simulink model "PV_with_boost_converter"  (R2018b)
settings: Solver=FixedStepDiscrete  StartTime=0.0  StopTime=3  RelTol=1e-3
undefined symbols (not defined in the file): L, sigbuilder_block
libraries: powerlib x11, re_lib x1, powerlib_meascontrol x1
settings Model: Creator=jetha  LastModifiedBy=jetha

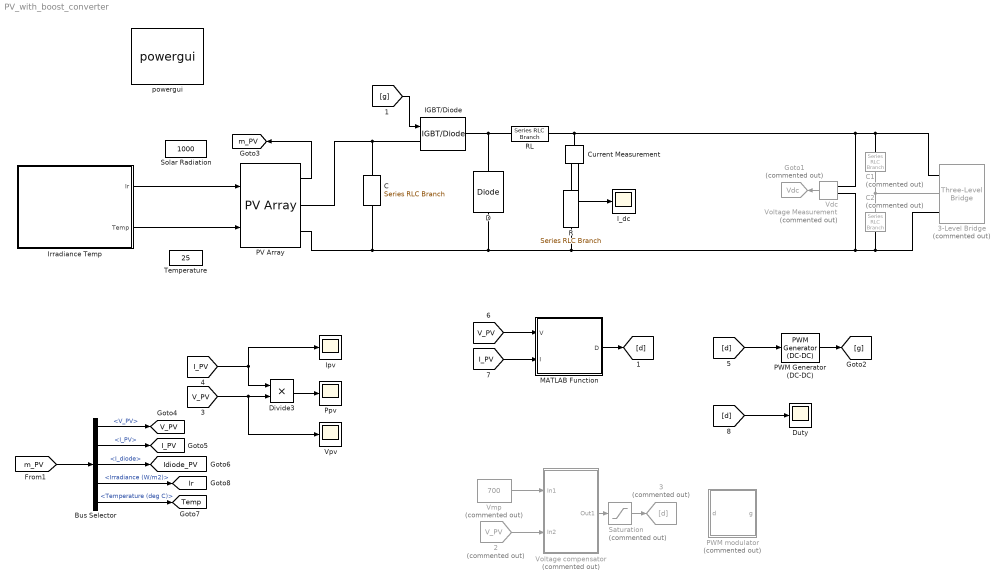
== system PV_with_boost_converter ==
  "       3" : Goto  Commented=on  GotoTag=d
  "   2" : From  Commented=on  GotoTag=V_PV  TagVisibility=global
      settings: CloseFcn=tagdialog Close
  3-Level Bridge : powerlib/Power Electronics/Three-Level Bridge  Commented=on  Arms=3  SnubberResistance=1e6  SbubberCapacitance=inf  Device=IGBT / Diodes  Ron=0.2e-3  ForwardVoltages="[  0  0 ]"  Measurements=None
      settings: SourceProductName=Simscape Electrical  SourceProductBaseCode=PS
  Bus Selector : BusSelector  OutputSignals=V_PV,I_PV,I_diode,Irradiance (W/m2),Temperature (deg C)
  C : powerlib/Elements/Series RLC Branch  LConnTagsString=__new0  RConnTagsString=__new0  BranchType=C  Resistance=1  Inductance=L  SetiL0=off  InitialCurrent=0  Capacitance=10e-3  Setx0=off  InitialVoltage=Vmp  Measurements=None
      settings: SourceProductName=Simscape Electrical
  C1 : powerlib/Elements/Series RLC Branch  Commented=on  LConnTagsString=__new0  RConnTagsString=__new0  BranchType=C  Resistance=1.0  Inductance=1.0  SetiL0=off  InitialCurrent=0  Capacitance=12e-3  Setx0=off  InitialVoltage=0  Measurements=None
      settings: SourceProductName=Simscape Electrical
  C2 : powerlib/Elements/Series RLC Branch  Commented=on  LConnTagsString=__new0  RConnTagsString=__new0  BranchType=C  Resistance=1.0  Inductance=1.0  SetiL0=off  InitialCurrent=0  Capacitance=12e-3  Setx0=off  InitialVoltage=0  Measurements=None
      settings: SourceProductName=Simscape Electrical
  Current Measurement : powerlib/Measurements/Current Measurement  PhasorSimulation=off  OutputType=Complex  PSBequivalent=0
  D : powerlib/Power Electronics/Diode  Ron=1e-4  Lon=0  Vf=0  IC=0  UseSnubber=off  Rs=inf  Cs=inf  Measurements=off
      settings: SourceProductName=Simscape Electrical
  Divide3 : Product  Inputs=**
  Duty : Scope
  Goto1 : Goto  Commented=on  GotoTag=Vdc  TagVisibility=global
  IGBT/Diode : powerlib/Power Electronics/IGBT//Diode  Ron=1e-3  Rs=1e5  Cs=inf  Measurements=off
  I_dc : Scope
  Ipv : Scope
  Irradiance Temp : Subsystem  Tag=STV Subsys  LoadFcn=sigbuilder_block('load');  StartFcn=sigbuilder_block('start');  StopFcn=sigbuilder_block('stop');  ClipboardFcn=sigbuilder_block('clipboard');  mask(Sigbuilder block){tuvar=[0:10]}
      mask help: Sigbuilder GUI
      mask init:
      | if ~strcmp(get_param(bdroot(gcbh),'SimulationStatus'),'stopped') tuvar = sigbuilder_block('maskInit'); end
      settings: CopyFcn=sigbuilder_block('copy');  DeleteFcn=sigbuilder_block('delete');  ModelCloseFcn=sigbuilder_block('modelClose');  PreSaveFcn=sigbuilder_block('preSave');  PauseFcn=sigbuilder_block('pause')  ContinueFcn=sigbuilder_block('continue')  NameChangeFcn=sigbuilder_block('namechange');  OpenFcn=sigbuilder_block('open',[216.75 153.75 550.5 395.25 ]);  CloseFcn=sigbuilder_block('close');
      mask Display: plot(0, 0, 100, 100,[2, 2, 32, 32, 2], [68, 8, 8, 68, 68],[32, 2], [38, 38], [32, 19, 2],[53, 60, 44], [32, 17, 17, 2],[16, 16, 31, 31]);txt = getActiveGroup(gcbh);text(2, 100, txt,'verticalAlignment', 'top');
  MATLAB Function : MATLAB Function  TreatAsAtomicUnit=on
  PV Array : re_lib/Solar/PV Array  Npar=4  Nser=20  PlotType=array @ 1000 W/m2 & specified temperatures  S_vec="[ 1000  500  100 ]"  Temp_C_vec="[ 25  50]"  ModuleName=Waaree Energies WSM-315  PlotWhenSelected=off  Pm=315  Ncell=72  Voc=43  Isc=9.77  Vm=35  Im=9  beta_Voc_pc=-0.338  alpha_Isc_pc=0.040901  beta_Voc=-0.14534  alpha_Isc=0.003996  IL=9.7966  I0=1.447e-10  nI=0.93356  Rsh=115.0566  Rs=0.31273  BAL=off  Tc=1e-6  Tfilter=5e-6
  PWM modulator : Subsystem  Commented=on
  PWM Generator (DC-DC) : powerlib_meascontrol/Pulse & Signal Generators/PWM Generator (DC-DC)  Fsw=10000  Ts=0
  Ppv : Scope
  R : powerlib/Elements/Series RLC Branch  LConnTagsString=__new0  RConnTagsString=__new0  BranchType=R  Resistance=5  Inductance=5e-3  SetiL0=off  InitialCurrent=0  Capacitance=1e-6  Setx0=off  InitialVoltage=0  Measurements=None
      settings: SourceProductName=Simscape Electrical
  RL : powerlib/Elements/Series RLC Branch  LConnTagsString=__new0  RConnTagsString=__new0  BranchType=RL  Resistance=5e-3  Inductance=10e-3  SetiL0=off  InitialCurrent=0  Capacitance=1e-6  Setx0=off  InitialVoltage=0  Measurements=None
      settings: SourceProductName=Simscape Electrical
  Saturation : Saturate  Commented=on  UpperLimit=1  LowerLimit=0
  Solar Radiation : Constant  Value=1000
  Temperature : Constant  Value=25
  "Vdc " : powerlib/Measurements/Voltage Measurement  Tag=PoWeRsYsTeMmEaSuReMeNt  Commented=on  PhasorSimulation=off  OutputType=Magnitude  PSBequivalent=0
      settings: SourceProductName=Simscape Electrical
  Vmp : Constant  Commented=on  Value=700
  Voltage compensator : Subsystem  Commented=on
  Vpv : Scope
  powergui : powerlib/powergui  Priority=1  SimulationMode=Discrete  SampleTime=5e-7  frequency=60  Iterations=50  frequencyindice=0  Pbase=100e6  ErrMax=1e-4  UnitsV=kV  UnitsW=MW  buscounter=0  FunctionMessages=off  echomessages=off  EnableUseOfTLC=off  CurrentSourceSwitches=off  DisableSnubberDevices=off  DisableRonSwitches=off  DisableVfSwitches=off  DisplayEquations=off  SolverType=Tustin/Backward Euler (TBE)  Interpol=off  ExternalGateDelay=off  methode=off  Ts=100  x0status=blocks  SPID=off  SwTol=0  HookPort=off  RestoreLinks=warning  ResistiveCurrentMeasurement=off  Frange=[0:2:500]  Ylog=off  Xlog=on  ShowGrid=off  save=off  variable=ZData  structure=0  ZoomFFT=off  StartTime=0.0  cycles=1  DisplayStyle=1  fundamental=60  FreqAxis=off  MaxFrequency=1000  frequencyindicesteady=1  RmsSteady=1  display=off
  tag scope: I_PV=global, Idiode_PV=global, Ir=global, Temp=global, V_PV=global, m_PV=global
  wires:
  Divide3/1 -> Ppv/1
  [I_PV] -> Ipv/1, Divide3/1
  [V_PV] -> Divide3/2, Vpv/1
  Voltage compensator/1(Out1) -> Saturation/1
  PWM Generator (DC-DC)/1 -> [g]
  "   2"/1 -> Voltage compensator/2(In2)
  [d] -> PWM Generator (DC-DC)/1
  PV Array/1 -> [m_PV]
  Bus Selector/3 -> [Idiode_PV]  "<I_diode>"
  Bus Selector/4 -> [Ir]  "<Irradiance (W/m2)>"
  Bus Selector/1 -> [V_PV]  "<V_PV>"
  Bus Selector/5 -> [Temp]  "<Temperature (deg C)>"
  Bus Selector/2 -> [I_PV]  "<I_PV>"
  [m_PV] -> Bus Selector/1
  "Vdc "/1 -> Goto1/1
  [g] -> IGBT/Diode/1
  Saturation/1 -> "       3"/1
  Current Measurement/1 -> I_dc/1
  [V_PV] -> MATLAB Function/1(V)
  [I_PV] -> MATLAB Function/2(I)
  MATLAB Function/1(D) -> [d]
  Vmp/1 -> Voltage compensator/1(In1)
  [d] -> Duty/1
  Irradiance Temp/1(Ir) -> PV Array/1
  Irradiance Temp/2(Temp) -> PV Array/2
  connections:
  C2/RConn1 -- 3-Level Bridge/RConn3 -- "Vdc "/LConn2 -- R/RConn1 -- C/RConn1 -- PV Array/RConn2 -- D/LConn1
  RL/LConn1 -- Current Measurement/LConn1 -- C1/LConn1 -- 3-Level Bridge/RConn1 -- "Vdc "/LConn1
  3-Level Bridge/RConn2 -- C1/RConn1 -- C2/LConn1
  R/LConn1 -- Current Measurement/RConn1
  D/RConn1 -- IGBT/Diode/RConn1 -- RL/RConn1
  PV Array/RConn1 -- C/LConn1 -- IGBT/Diode/LConn1

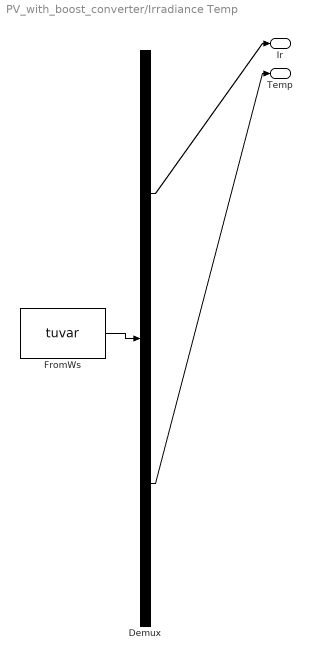
== system PV_with_boost_converter/Irradiance Temp ==
  Demux : Demux  Tag=STV Demux  Outputs=2
  FromWs : FromWorkspace  Tag=STV FromWs  VariableName=tuvar  SampleTime=0
      SigBuilderData=|
      | common.afterFinalStr = 'Extrapolate'
      | common.sampleTime = '0'
      | dataSet(1).timeRange = [0 1]
      | dataSet(1).name = 'Constant Irradiance'
      | dataSet(2).timeRange = [0 1]
      | dataSet(2).name = 'Step Irradiance'
      | dataSet(3).timeRange = [0 3]
      | dataSet(3).name = 'Ramp-up/down Irradiance'
      | sbobj.Groups(1).Name = 'Constant Irradiance'
      | sbobj.Groups(1).Signals(1).Name = 'Ir'
      | sbobj.Groups(1).Signals(1).XData = [0 1]
      | sbobj.Groups(1).Signals(1).YData = [1000 1000]
      | sbobj.Groups(1).Signals(2).Name = 'Temp'
      | sbobj.Groups(1).Signals(2).XData = [0 1 1 2]
      | sbobj.Groups(1).Signals(2).YData = [0 0 1 1]
      | sbobj.Groups(1).TimeRange = [0 1]
      | sbobj.Groups(2).Name = 'Step Irradiance'
      | sbobj.Groups(2).Signals(1).Name = 'Ir'
      | sbobj.Groups(2).Signals(1).XData = [0 0.252 0.252 1]
      | sbobj.Groups(2).Signals(1).YData = [600 600 1000 1000]
      | sbobj.Groups(2).Signals(2).Name = 'Temp'
      | sbobj.Groups(2).Signals(2).XData = [0 1 1 2]
      | sbobj.Groups(2).Signals(2).YData = [0 0 1 1]
      | sbobj.Groups(2).TimeRange = [0 1]
      | sbobj.Groups(3).Name = 'Ramp-up/down Irradiance'
      | sbobj.Groups(3).Signals(1).Name = 'Ir'
      | sbobj.Groups(3).Signals(1).XData = [0 0.6 1.1 1.2 1.7 3]
      | sbobj.Groups(3).Signals(1).YData = [1000 1000 250 250 1000 1000]
      | sbobj.Groups(3).Signals(2).Name = 'Temp'
      | sbobj.Groups(3).Signals(2).XData = [0 2 2.1 3]
      | sbobj.Groups(3).Signals(2).YData = [25 25 50 50]
      | sbobj.Groups(3).TimeRange = [0 3]
  Ir : Outport  Tag=STV Outport
  Temp : Outport  Tag=STV Outport  Port=2
  wires:
  Demux/1 -> Ir/1
  FromWs/1 -> Demux/1
  Demux/2 -> Temp/1

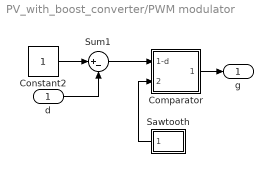
== system PV_with_boost_converter/PWM modulator ==
  d : Inport
  Comparator : Subsystem
      settings: RTWSystemCode=Inline
  Constant2 : Constant
  Sawtooth : Subsystem
  Sum1 : Sum  Inputs=|+-
  g : Outport
  wires:
  Sawtooth/1(Out1) -> Comparator/2(Sawtooth)
  Constant2/1 -> Sum1/1
  Sum1/1 -> Comparator/1(1-d)
  Comparator/1(Out1) -> g/1
  d/1 -> Sum1/2

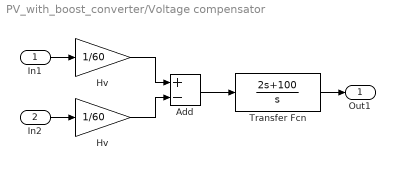
== system PV_with_boost_converter/Voltage compensator ==
  In1 : Inport
  In2 : Inport  Port=2
  Add : Sum  Inputs=+-
  Hv : Gain  Gain=1/60
  "Hv " : Gain  Gain=1/60
  Transfer Fcn : TransferFcn  Numerator=[2 100]  Denominator=[1 0]
  Out1 : Outport
  wires:
  "Hv "/1 -> Add/1
  Hv/1 -> Add/2
  Add/1 -> Transfer Fcn/1
  In1/1 -> "Hv "/1
  Transfer Fcn/1 -> Out1/1
  In2/1 -> Hv/1

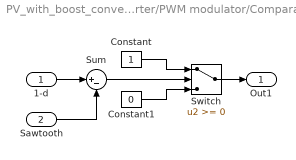
== system PV_with_boost_converter/PWM modulator/Comparator ==
  1-d : Inport
  Sawtooth : Inport  Port=2
  Constant : Constant
  Constant1 : Constant  Value=0
  Sum : Sum  Inputs=|+-
  Switch : Switch
  Out1 : Outport
  wires:
  Constant1/1 -> Switch/3
  Constant/1 -> Switch/1
  Sum/1 -> Switch/2
  1-d/1 -> Sum/1
  Switch/1 -> Out1/1
  Sawtooth/1 -> Sum/2

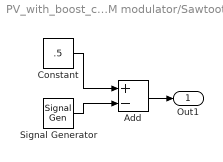
== system PV_with_boost_converter/PWM modulator/Sawtooth ==
  Add : Sum  Inputs=+-
  Constant : Constant  Value=.5
  Signal Generator : SignalGenerator  WaveForm=sawtooth  Amplitude=.5  Frequency=10000
  Out1 : Outport
  wires:
  Constant/1 -> Add/1
  Signal Generator/1 -> Add/2
  Add/1 -> Out1/1

== matlab function PV_with_boost_converter/MATLAB Function ==
  data: V input; D output; I input
function D = MPPT(V, I)

persistent Dold Pold Vold

if isempty(Vold)
    Dold = 0.8;
    Pold = 0;
    Vold = 0;
end

deltaD = 0.00001;

P = V * I;
dV = V - Vold;
dP = P - Pold;

if dP ~= 0
    if dP > 0
        if dV > 0
            D = Dold - deltaD;
        else
            D = Dold + deltaD;
        end
    else
        if dV < 0
            D = Dold - deltaD;
        else
            D = Dold + deltaD;
        end    
    end
else
    D=Dold;
end

if D >= 1 || D<= 0
    D=Dold;
end

Dold=D;
Vold=V;
Pold=P;
